simulink model "single_integrator"  (R2020b)
settings: Solver=VariableStepAuto  StartTime=0.0  StopTime=10.0  RelTol=1e-3
values from neighbouring files (symbols this model uses):
  Current_coordinates = [Prev_Px(i); Prev_Py(i)]    [lloyd_wtd_heterogeneous.m]    (also in lloyd_wtd_heterogeneous_adaptive.m)
  Target_coordinates = [Px(i);Py(i)]    [lloyd_wtd_heterogeneous.m]    (also in lloyd_wtd_heterogeneous_adaptive.m)
libraries: simulink x1
settings Model: Creator=nijil  LastModifiedBy=nijil

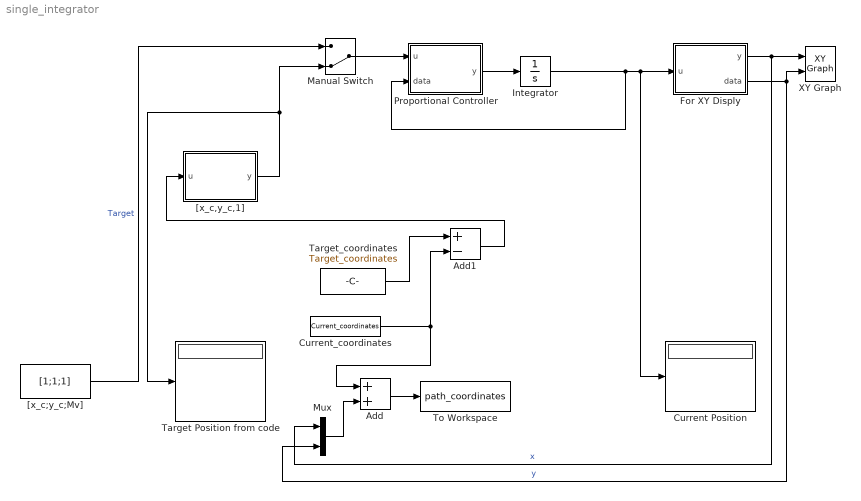
== system single_integrator ==
  Add : Sum
  Add1 : Sum  Inputs=+-
  Current Position : Display
  Current_coordinates : Constant  Value=Current_coordinates
  For XY Disply : MATLAB Function  TreatAsAtomicUnit=on
  Integrator : Integrator  InitialCondition=[0 0]
  Manual Switch : ManualSwitch  CurrentSetting=0
  Mux : Mux  Inputs=2
  Proportional Controller : MATLAB Function  TreatAsAtomicUnit=on
  Target Position from code : Display
  Target_coordinates : Constant  Value=Target_coordinates
  To Workspace : ToWorkspace  VariableName=path_coordinates  SaveFormat=Timeseries  SampleTime=-1
  XY Graph : simulink/Sinks/XY Graph  xmin=-10  xmax=10  ymin=-10  ymax=10  st=-1
  "[x_c,y_c,1]" : MATLAB Function  TreatAsAtomicUnit=on
  "[x_c;y_c;Mv]" : Constant  Value=[1;1;1]
  wires:
  "[x_c,y_c,1]"/1(y) -> Target Position from code/1, Manual Switch/2
  "[x_c;y_c;Mv]"/1 -> Manual Switch/1  "Target"
  Add1/1 -> "[x_c,y_c,1]"/1(u)
  Add/1 -> To Workspace/1
  For XY Disply/1(y) -> XY Graph/1, Mux/1  "x"
  Current_coordinates/1 -> Add1/2, Add/1
  For XY Disply/2(data) -> XY Graph/2, Mux/2  "y"
  Mux/1 -> Add/2
  Target_coordinates/1 -> Add1/1
  Proportional Controller/1(y) -> Integrator/1
  Manual Switch/1 -> Proportional Controller/1(u)
  Integrator/1 -> For XY Disply/1(u), Current Position/1, Proportional Controller/2(data)

== matlab function single_integrator/Proportional Controller ==
  data: u input; y output; data input
function y = fcn(u, data)
%u=(xc,yc) data=(x,y)
k=6;
y =k*[u(1)-data(1) u(2)-data(2)] ;

== matlab function single_integrator/For XY Disply ==
  data: u input; y output; data output
function [y,data] = fcn(u)
y=u(1);
data = u(2);

== matlab function single_integrator/[x_c,y_c,1] ==
  data: u input; y output
function y = fcn(u)

y = [u(1),u(2),1];
